simulink model "motorSim"  (R2017b)
settings: Solver=FixedStepAuto  StartTime=0.0  StopTime=25.0  FixedStep=0.01  RelTol=1e-3
undefined symbols (not defined in the file or in its folder): gain, pole
settings Model: Creator=aaten  LastModifiedBy=aaten

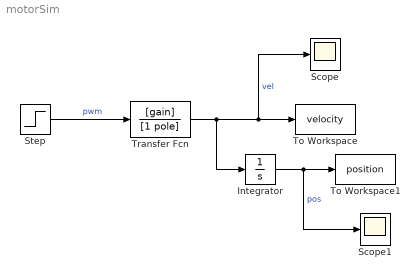
== system motorSim ==
  Integrator : Integrator
  Scope : Scope
  Scope1 : Scope
  Step : Step  Time=0  After=gain(1)  SampleTime=0
  To Workspace : ToWorkspace  VariableName=velocity  SaveFormat=Timeseries  SampleTime=-1
  To Workspace1 : ToWorkspace  VariableName=position  SaveFormat=Timeseries  SampleTime=-1
  Transfer Fcn : TransferFcn  Numerator=[gain]  Denominator=[1 pole]
  wires:
  Step/1 -> Transfer Fcn/1  "pwm"
  Transfer Fcn/1 -> Scope/1, To Workspace/1, Integrator/1  "vel"
  Integrator/1 -> Scope1/1, To Workspace1/1  "pos"
